simulink model "Modular_Model_New_Board"  (R2018a)
settings: Solver=FixedStepAuto  StartTime=0.0  StopTime=Tfinal  FixedStep=SampleTime*1e-2  MinStep=SampleTime*1e-2  RelTol=1e-3
values from neighbouring files (symbols this model uses):
  ESRA = 21.1e-3    (= 0.0211)    [sim_param_new_board.m]
  ESRB = 21.1e-3    (= 0.0211)    [sim_param_new_board.m]
  ESRC = 21.1e-3    (= 0.0211)    [sim_param_new_board.m]
  ffund = 50    [sim_param_new_board.m]
  LAMid = 01.30e-9    (= 1.3e-09)    [sim_param_new_board.m]
  LBMid = 01.30e-9    (= 1.3e-09)    [sim_param_new_board.m]
  LCMid = 01.30e-9    (= 1.3e-09)    [sim_param_new_board.m]
  ModulationIndex1 = 0.9    [sim_param_new_board.m]
  Module1Phase = 0    [sim_param_new_board.m]
  RABBot = 10.20e-9    (= 1.02e-08)    [sim_param_new_board.m]
  RABot = 20.25e-9    (= 2.025e-08)    [sim_param_new_board.m]
  RABTop = 18.30e-9    (= 1.83e-08)    [sim_param_new_board.m]
  RAMid = 01.30e-9    (= 1.3e-09)    [sim_param_new_board.m]
  RATop = 03.40e-9    (= 3.4e-09)    [sim_param_new_board.m]
  RBBot = 20.38e-9    (= 2.038e-08)    [sim_param_new_board.m]
  RBCBot = 11.14e-9    (= 1.114e-08)    [sim_param_new_board.m]
  RBCTop = 21.84e-9    (= 2.184e-08)    [sim_param_new_board.m]
  RBMid = 01.30e-9    (= 1.3e-09)    [sim_param_new_board.m]
  RBTop = 03.38e-9    (= 3.38e-09)    [sim_param_new_board.m]
  RCBot = 20.94e-9    (= 2.094e-08)    [sim_param_new_board.m]
  RCMid = 01.30e-9    (= 1.3e-09)    [sim_param_new_board.m]
  RCTop = 03.41e-9    (= 3.41e-09)    [sim_param_new_board.m]
  Rin = 0.1    [sim_param_new_board.m]
  Rload1 = Z1*PF    [sim_param_new_board.m]
  Vmodule = 270    [sim_param_new_board.m]
  VpulseMax = 6    [sim_param_new_board.m]
  VpulseMin = -3    [sim_param_new_board.m]
libraries: elec_lib x81, fl_lib x38, nesl_utility x38, simulink x12, powerlib_meascontrol x4
(part 3 of 3)

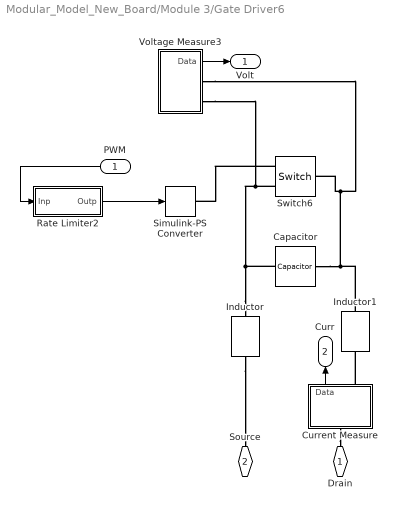
== system Modular_Model_New_Board/Module 3/Gate Driver6 ==
  PWM : Inport
  Capacitor : elec_lib/Passive Devices/Capacitor  enable_table=0  c=142e-12 F  Cvec=[1e-05, 1e-06] F  Vvec=[0, 10] V  CV_table_symmetry=1  C_tol=5  enable_C_tol=0  tol_distribution=1  nSigma=4  r=1e-6 Ohm  g=0 1/Ohm  enable_operating_limits=0  operating_limit_action=2  max_working_voltage_range=[-25, 25] V  power_rating=1 W  enable_faults=0  fault_action=1  Cscale_faulted=100  R_faulted=1e-3 Ohm  G_faulted=0 1/Ohm  tau_fault=1e-3 s  enable_temporal_fault=0  t_fault=1 s  enable_behavioral_fault=0  max_permissible_voltage_range=[-100, 100] V  t_fail_on_voltage=1 s  i_specify=off  i_priority=None  i=0 A  i_nominal_specify=off  i_nominal_unit=A  i_nominal_value=1  v_specify=off  v_priority=None  v=0 V  v_nominal_specify=off  v_nominal_unit=V  v_nominal_value=1  vc_specify=on  vc_priority=High  vc=0 V  vc_nominal_specify=off  vc_nominal_unit=V  vc_nominal_value=1
  Current Measure : Subsystem
  Inductor : elec_lib/Passive Devices/Inductor  l=Ls H  L_tol=20  enable_L_tol=0  tol_distribution=1  nSigma=4  r=0 Ohm  g=1e-9 1/Ohm  enable_operating_limits=0  operating_limit_action=2  max_working_current=1 A  power_rating=1 W  enable_faults=0  fault_action=1  lambdaPercent=50  k_faulted=0.9999  turnsShort=0  openCct=0  groundShort=0  groundShortG=0 1/Ohm  tau_fault=1e-3 s  enable_temporal_fault=0  t_fault=1 s  enable_behavioral_fault=0  max_permissible_voltage=100 V  n_fail_on_voltage=1  max_permissible_current=1 A  t_fail_on_current=1 s  i_L_specify=on  i_L_priority=High  i_L=0 A  i_L_nominal_specify=off  i_L_nominal_unit=A  i_L_nominal_value=1
      settings: SourceProductName=Simscape Electronics  SourceProductBaseCode=SN
  Inductor1 : elec_lib/Passive Devices/Inductor  l=Ld H  L_tol=20  enable_L_tol=0  tol_distribution=1  nSigma=4  r=0 Ohm  g=1e-9 1/Ohm  enable_operating_limits=0  operating_limit_action=2  max_working_current=1 A  power_rating=1 W  enable_faults=0  fault_action=1  lambdaPercent=50  k_faulted=0.9999  turnsShort=0  openCct=0  groundShort=0  groundShortG=0 1/Ohm  tau_fault=1e-3 s  enable_temporal_fault=0  t_fault=1 s  enable_behavioral_fault=0  max_permissible_voltage=100 V  n_fail_on_voltage=1  max_permissible_current=1 A  t_fail_on_current=1 s  i_L_specify=on  i_L_priority=High  i_L=0 A  i_L_nominal_specify=off  i_L_nominal_unit=A  i_L_nominal_value=1
      settings: SourceProductName=Simscape Electronics  SourceProductBaseCode=SN
  Rate Limiter2 : Subsystem
  Simulink-PS Converter : nesl_utility/Simulink-PS Converter  PhysicalDomain=network_engine_domain  SubClassName=ps_input  LeftPortType=input  RightPortType=output  PseudoPeriodic=off  Frequencies=[]  NoiseDistribution=none  NoiseParameters=[]  Unit=1  AffineConversion=off  FilteringAndDerivatives=zero  SimscapeFilterOrder=1  InputFilterTimeConstant=0.001  UdotUserProvided=1
  Switch6 : fl_lib/Electrical/Electrical Elements/Switch  R_closed=0.05 Ohm  G_open=1e-8 1/Ohm  Threshold=1.7  i_specify=off  i_priority=None  i=0 A  i_nominal_specify=off  i_nominal_unit=A  i_nominal_value=1  v_specify=off  v_priority=None  v=0 V  v_nominal_specify=off  v_nominal_unit=V  v_nominal_value=1
      settings: SourceProductName=Simscape
  Voltage Measure3 : Subsystem
  Drain : PMIOPort  Side=Left
  Source : PMIOPort  Port=2  Side=Left
  Volt : Outport
  Curr : Outport  Port=2
  wires:
  PWM/1 -> Rate Limiter2/1(Inp)
  Rate Limiter2/1(Outp) -> Simulink-PS Converter/1
  Voltage Measure3/1(Data) -> Volt/1
  Current Measure/1(Data) -> Curr/1
  connections:
  Switch6/RConn1 -- Simulink-PS Converter/RConn1
  Inductor/LConn1 -- Voltage Measure3/RConn2 -- Switch6/RConn2 -- Capacitor/RConn1
  Voltage Measure3/RConn1 -- Switch6/LConn1 -- Capacitor/LConn1 -- Inductor1/LConn1
  Current Measure/LConn1 -- Drain/RConn1
  Inductor/RConn1 -- Source/RConn1
  Current Measure/RConn1 -- Inductor1/RConn1

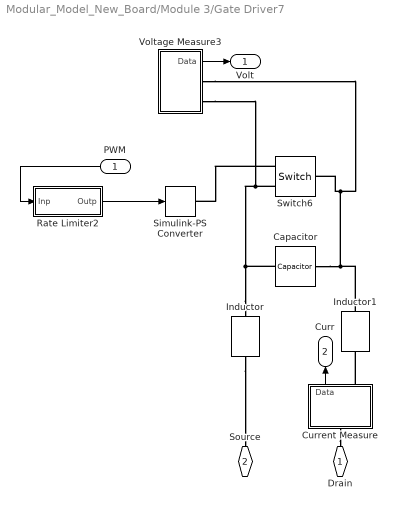
== system Modular_Model_New_Board/Module 3/Gate Driver7 ==
  PWM : Inport
  Capacitor : elec_lib/Passive Devices/Capacitor  enable_table=0  c=142e-12 F  Cvec=[1e-05, 1e-06] F  Vvec=[0, 10] V  CV_table_symmetry=1  C_tol=5  enable_C_tol=0  tol_distribution=1  nSigma=4  r=1e-6 Ohm  g=0 1/Ohm  enable_operating_limits=0  operating_limit_action=2  max_working_voltage_range=[-25, 25] V  power_rating=1 W  enable_faults=0  fault_action=1  Cscale_faulted=100  R_faulted=1e-3 Ohm  G_faulted=0 1/Ohm  tau_fault=1e-3 s  enable_temporal_fault=0  t_fault=1 s  enable_behavioral_fault=0  max_permissible_voltage_range=[-100, 100] V  t_fail_on_voltage=1 s  i_specify=off  i_priority=None  i=0 A  i_nominal_specify=off  i_nominal_unit=A  i_nominal_value=1  v_specify=off  v_priority=None  v=0 V  v_nominal_specify=off  v_nominal_unit=V  v_nominal_value=1  vc_specify=on  vc_priority=High  vc=0 V  vc_nominal_specify=off  vc_nominal_unit=V  vc_nominal_value=1
  Current Measure : Subsystem
  Inductor : elec_lib/Passive Devices/Inductor  l=Ls H  L_tol=20  enable_L_tol=0  tol_distribution=1  nSigma=4  r=0 Ohm  g=1e-9 1/Ohm  enable_operating_limits=0  operating_limit_action=2  max_working_current=1 A  power_rating=1 W  enable_faults=0  fault_action=1  lambdaPercent=50  k_faulted=0.9999  turnsShort=0  openCct=0  groundShort=0  groundShortG=0 1/Ohm  tau_fault=1e-3 s  enable_temporal_fault=0  t_fault=1 s  enable_behavioral_fault=0  max_permissible_voltage=100 V  n_fail_on_voltage=1  max_permissible_current=1 A  t_fail_on_current=1 s  i_L_specify=on  i_L_priority=High  i_L=0 A  i_L_nominal_specify=off  i_L_nominal_unit=A  i_L_nominal_value=1
      settings: SourceProductName=Simscape Electronics  SourceProductBaseCode=SN
  Inductor1 : elec_lib/Passive Devices/Inductor  l=Ld H  L_tol=20  enable_L_tol=0  tol_distribution=1  nSigma=4  r=0 Ohm  g=1e-9 1/Ohm  enable_operating_limits=0  operating_limit_action=2  max_working_current=1 A  power_rating=1 W  enable_faults=0  fault_action=1  lambdaPercent=50  k_faulted=0.9999  turnsShort=0  openCct=0  groundShort=0  groundShortG=0 1/Ohm  tau_fault=1e-3 s  enable_temporal_fault=0  t_fault=1 s  enable_behavioral_fault=0  max_permissible_voltage=100 V  n_fail_on_voltage=1  max_permissible_current=1 A  t_fail_on_current=1 s  i_L_specify=on  i_L_priority=High  i_L=0 A  i_L_nominal_specify=off  i_L_nominal_unit=A  i_L_nominal_value=1
      settings: SourceProductName=Simscape Electronics  SourceProductBaseCode=SN
  Rate Limiter2 : Subsystem
  Simulink-PS Converter : nesl_utility/Simulink-PS Converter  PhysicalDomain=network_engine_domain  SubClassName=ps_input  LeftPortType=input  RightPortType=output  PseudoPeriodic=off  Frequencies=[]  NoiseDistribution=none  NoiseParameters=[]  Unit=1  AffineConversion=off  FilteringAndDerivatives=zero  SimscapeFilterOrder=1  InputFilterTimeConstant=0.001  UdotUserProvided=1
  Switch6 : fl_lib/Electrical/Electrical Elements/Switch  R_closed=0.05 Ohm  G_open=1e-8 1/Ohm  Threshold=1.7  i_specify=off  i_priority=None  i=0 A  i_nominal_specify=off  i_nominal_unit=A  i_nominal_value=1  v_specify=off  v_priority=None  v=0 V  v_nominal_specify=off  v_nominal_unit=V  v_nominal_value=1
      settings: SourceProductName=Simscape
  Voltage Measure3 : Subsystem
  Drain : PMIOPort  Side=Left
  Source : PMIOPort  Port=2  Side=Left
  Volt : Outport
  Curr : Outport  Port=2
  wires:
  PWM/1 -> Rate Limiter2/1(Inp)
  Rate Limiter2/1(Outp) -> Simulink-PS Converter/1
  Voltage Measure3/1(Data) -> Volt/1
  Current Measure/1(Data) -> Curr/1
  connections:
  Switch6/RConn1 -- Simulink-PS Converter/RConn1
  Inductor/LConn1 -- Voltage Measure3/RConn2 -- Switch6/RConn2 -- Capacitor/RConn1
  Voltage Measure3/RConn1 -- Switch6/LConn1 -- Capacitor/LConn1 -- Inductor1/LConn1
  Current Measure/LConn1 -- Drain/RConn1
  Inductor/RConn1 -- Source/RConn1
  Current Measure/RConn1 -- Inductor1/RConn1

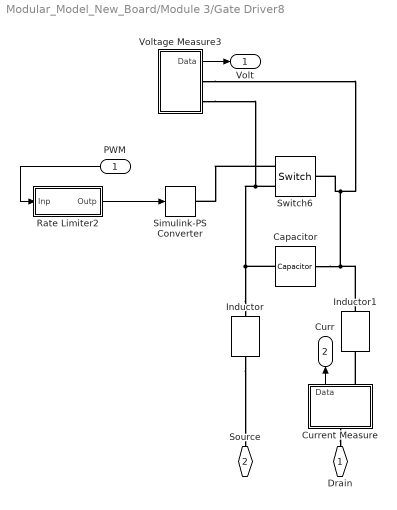
== system Modular_Model_New_Board/Module 3/Gate Driver8 ==
  PWM : Inport
  Capacitor : elec_lib/Passive Devices/Capacitor  enable_table=0  c=142e-12 F  Cvec=[1e-05, 1e-06] F  Vvec=[0, 10] V  CV_table_symmetry=1  C_tol=5  enable_C_tol=0  tol_distribution=1  nSigma=4  r=1e-6 Ohm  g=0 1/Ohm  enable_operating_limits=0  operating_limit_action=2  max_working_voltage_range=[-25, 25] V  power_rating=1 W  enable_faults=0  fault_action=1  Cscale_faulted=100  R_faulted=1e-3 Ohm  G_faulted=0 1/Ohm  tau_fault=1e-3 s  enable_temporal_fault=0  t_fault=1 s  enable_behavioral_fault=0  max_permissible_voltage_range=[-100, 100] V  t_fail_on_voltage=1 s  i_specify=off  i_priority=None  i=0 A  i_nominal_specify=off  i_nominal_unit=A  i_nominal_value=1  v_specify=off  v_priority=None  v=0 V  v_nominal_specify=off  v_nominal_unit=V  v_nominal_value=1  vc_specify=on  vc_priority=High  vc=0 V  vc_nominal_specify=off  vc_nominal_unit=V  vc_nominal_value=1
  Current Measure : Subsystem
  Inductor : elec_lib/Passive Devices/Inductor  l=Ls H  L_tol=20  enable_L_tol=0  tol_distribution=1  nSigma=4  r=0 Ohm  g=1e-9 1/Ohm  enable_operating_limits=0  operating_limit_action=2  max_working_current=1 A  power_rating=1 W  enable_faults=0  fault_action=1  lambdaPercent=50  k_faulted=0.9999  turnsShort=0  openCct=0  groundShort=0  groundShortG=0 1/Ohm  tau_fault=1e-3 s  enable_temporal_fault=0  t_fault=1 s  enable_behavioral_fault=0  max_permissible_voltage=100 V  n_fail_on_voltage=1  max_permissible_current=1 A  t_fail_on_current=1 s  i_L_specify=on  i_L_priority=High  i_L=0 A  i_L_nominal_specify=off  i_L_nominal_unit=A  i_L_nominal_value=1
      settings: SourceProductName=Simscape Electronics  SourceProductBaseCode=SN
  Inductor1 : elec_lib/Passive Devices/Inductor  l=Ld H  L_tol=20  enable_L_tol=0  tol_distribution=1  nSigma=4  r=0 Ohm  g=1e-9 1/Ohm  enable_operating_limits=0  operating_limit_action=2  max_working_current=1 A  power_rating=1 W  enable_faults=0  fault_action=1  lambdaPercent=50  k_faulted=0.9999  turnsShort=0  openCct=0  groundShort=0  groundShortG=0 1/Ohm  tau_fault=1e-3 s  enable_temporal_fault=0  t_fault=1 s  enable_behavioral_fault=0  max_permissible_voltage=100 V  n_fail_on_voltage=1  max_permissible_current=1 A  t_fail_on_current=1 s  i_L_specify=on  i_L_priority=High  i_L=0 A  i_L_nominal_specify=off  i_L_nominal_unit=A  i_L_nominal_value=1
      settings: SourceProductName=Simscape Electronics  SourceProductBaseCode=SN
  Rate Limiter2 : Subsystem
  Simulink-PS Converter : nesl_utility/Simulink-PS Converter  PhysicalDomain=network_engine_domain  SubClassName=ps_input  LeftPortType=input  RightPortType=output  PseudoPeriodic=off  Frequencies=[]  NoiseDistribution=none  NoiseParameters=[]  Unit=1  AffineConversion=off  FilteringAndDerivatives=zero  SimscapeFilterOrder=1  InputFilterTimeConstant=0.001  UdotUserProvided=1
  Switch6 : fl_lib/Electrical/Electrical Elements/Switch  R_closed=0.05 Ohm  G_open=1e-8 1/Ohm  Threshold=1.7  i_specify=off  i_priority=None  i=0 A  i_nominal_specify=off  i_nominal_unit=A  i_nominal_value=1  v_specify=off  v_priority=None  v=0 V  v_nominal_specify=off  v_nominal_unit=V  v_nominal_value=1
      settings: SourceProductName=Simscape
  Voltage Measure3 : Subsystem
  Drain : PMIOPort  Side=Left
  Source : PMIOPort  Port=2  Side=Left
  Volt : Outport
  Curr : Outport  Port=2
  wires:
  PWM/1 -> Rate Limiter2/1(Inp)
  Rate Limiter2/1(Outp) -> Simulink-PS Converter/1
  Voltage Measure3/1(Data) -> Volt/1
  Current Measure/1(Data) -> Curr/1
  connections:
  Switch6/RConn1 -- Simulink-PS Converter/RConn1
  Inductor/LConn1 -- Voltage Measure3/RConn2 -- Switch6/RConn2 -- Capacitor/RConn1
  Voltage Measure3/RConn1 -- Switch6/LConn1 -- Capacitor/LConn1 -- Inductor1/LConn1
  Current Measure/LConn1 -- Drain/RConn1
  Inductor/RConn1 -- Source/RConn1
  Current Measure/RConn1 -- Inductor1/RConn1

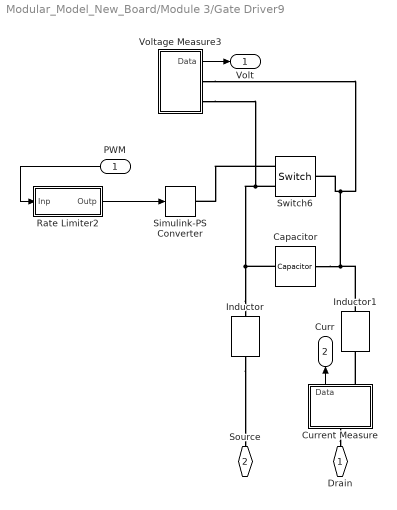
== system Modular_Model_New_Board/Module 3/Gate Driver9 ==
  PWM : Inport
  Capacitor : elec_lib/Passive Devices/Capacitor  enable_table=0  c=142e-12 F  Cvec=[1e-05, 1e-06] F  Vvec=[0, 10] V  CV_table_symmetry=1  C_tol=5  enable_C_tol=0  tol_distribution=1  nSigma=4  r=1e-6 Ohm  g=0 1/Ohm  enable_operating_limits=0  operating_limit_action=2  max_working_voltage_range=[-25, 25] V  power_rating=1 W  enable_faults=0  fault_action=1  Cscale_faulted=100  R_faulted=1e-3 Ohm  G_faulted=0 1/Ohm  tau_fault=1e-3 s  enable_temporal_fault=0  t_fault=1 s  enable_behavioral_fault=0  max_permissible_voltage_range=[-100, 100] V  t_fail_on_voltage=1 s  i_specify=off  i_priority=None  i=0 A  i_nominal_specify=off  i_nominal_unit=A  i_nominal_value=1  v_specify=off  v_priority=None  v=0 V  v_nominal_specify=off  v_nominal_unit=V  v_nominal_value=1  vc_specify=on  vc_priority=High  vc=0 V  vc_nominal_specify=off  vc_nominal_unit=V  vc_nominal_value=1
  Current Measure : Subsystem
  Inductor : elec_lib/Passive Devices/Inductor  l=Ls H  L_tol=20  enable_L_tol=0  tol_distribution=1  nSigma=4  r=0 Ohm  g=1e-9 1/Ohm  enable_operating_limits=0  operating_limit_action=2  max_working_current=1 A  power_rating=1 W  enable_faults=0  fault_action=1  lambdaPercent=50  k_faulted=0.9999  turnsShort=0  openCct=0  groundShort=0  groundShortG=0 1/Ohm  tau_fault=1e-3 s  enable_temporal_fault=0  t_fault=1 s  enable_behavioral_fault=0  max_permissible_voltage=100 V  n_fail_on_voltage=1  max_permissible_current=1 A  t_fail_on_current=1 s  i_L_specify=on  i_L_priority=High  i_L=0 A  i_L_nominal_specify=off  i_L_nominal_unit=A  i_L_nominal_value=1
      settings: SourceProductName=Simscape Electronics  SourceProductBaseCode=SN
  Inductor1 : elec_lib/Passive Devices/Inductor  l=Ld H  L_tol=20  enable_L_tol=0  tol_distribution=1  nSigma=4  r=0 Ohm  g=1e-9 1/Ohm  enable_operating_limits=0  operating_limit_action=2  max_working_current=1 A  power_rating=1 W  enable_faults=0  fault_action=1  lambdaPercent=50  k_faulted=0.9999  turnsShort=0  openCct=0  groundShort=0  groundShortG=0 1/Ohm  tau_fault=1e-3 s  enable_temporal_fault=0  t_fault=1 s  enable_behavioral_fault=0  max_permissible_voltage=100 V  n_fail_on_voltage=1  max_permissible_current=1 A  t_fail_on_current=1 s  i_L_specify=on  i_L_priority=High  i_L=0 A  i_L_nominal_specify=off  i_L_nominal_unit=A  i_L_nominal_value=1
      settings: SourceProductName=Simscape Electronics  SourceProductBaseCode=SN
  Rate Limiter2 : Subsystem
  Simulink-PS Converter : nesl_utility/Simulink-PS Converter  PhysicalDomain=network_engine_domain  SubClassName=ps_input  LeftPortType=input  RightPortType=output  PseudoPeriodic=off  Frequencies=[]  NoiseDistribution=none  NoiseParameters=[]  Unit=1  AffineConversion=off  FilteringAndDerivatives=zero  SimscapeFilterOrder=1  InputFilterTimeConstant=0.001  UdotUserProvided=1
  Switch6 : fl_lib/Electrical/Electrical Elements/Switch  R_closed=0.05 Ohm  G_open=1e-8 1/Ohm  Threshold=1.7  i_specify=off  i_priority=None  i=0 A  i_nominal_specify=off  i_nominal_unit=A  i_nominal_value=1  v_specify=off  v_priority=None  v=0 V  v_nominal_specify=off  v_nominal_unit=V  v_nominal_value=1
      settings: SourceProductName=Simscape
  Voltage Measure3 : Subsystem
  Drain : PMIOPort  Side=Left
  Source : PMIOPort  Port=2  Side=Left
  Volt : Outport
  Curr : Outport  Port=2
  wires:
  PWM/1 -> Rate Limiter2/1(Inp)
  Rate Limiter2/1(Outp) -> Simulink-PS Converter/1
  Voltage Measure3/1(Data) -> Volt/1
  Current Measure/1(Data) -> Curr/1
  connections:
  Switch6/RConn1 -- Simulink-PS Converter/RConn1
  Inductor/LConn1 -- Voltage Measure3/RConn2 -- Switch6/RConn2 -- Capacitor/RConn1
  Voltage Measure3/RConn1 -- Switch6/LConn1 -- Capacitor/LConn1 -- Inductor1/LConn1
  Current Measure/LConn1 -- Drain/RConn1
  Inductor/RConn1 -- Source/RConn1
  Current Measure/RConn1 -- Inductor1/RConn1

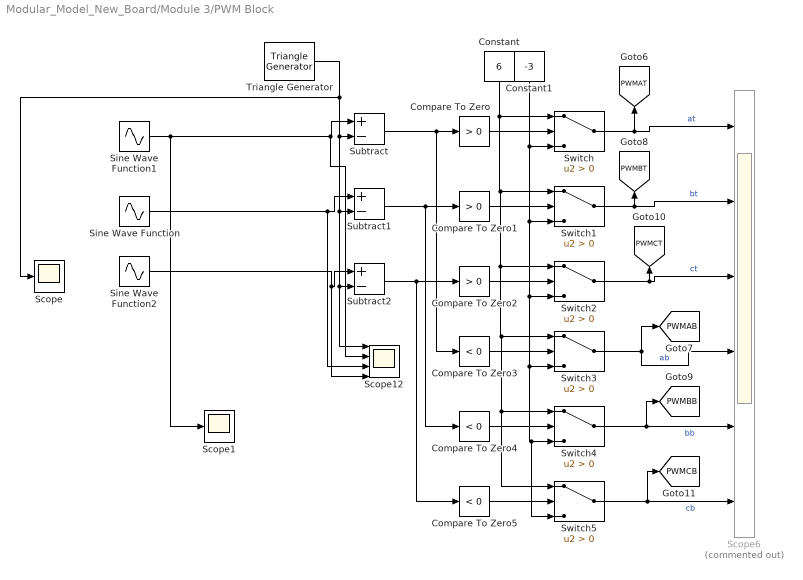
== system Modular_Model_New_Board/Module 3/PWM Block ==
  Compare To Zero : simulink/Logic and Bit Operations/Compare To Zero  relop=>  OutDataTypeStr=boolean
  Compare To Zero1 : simulink/Logic and Bit Operations/Compare To Zero  relop=>  OutDataTypeStr=boolean
  Compare To Zero2 : simulink/Logic and Bit Operations/Compare To Zero  relop=>  OutDataTypeStr=boolean
  Compare To Zero3 : simulink/Logic and Bit Operations/Compare To Zero  relop=<  OutDataTypeStr=boolean
  Compare To Zero4 : simulink/Logic and Bit Operations/Compare To Zero  relop=<  OutDataTypeStr=boolean
  Compare To Zero5 : simulink/Logic and Bit Operations/Compare To Zero  relop=<  OutDataTypeStr=boolean
  Constant : Constant  Value=6
  Constant1 : Constant  Value=-3
  Scope : Scope
  Scope1 : Scope
  Scope12 : Scope  NumInputPorts=4
  Scope6 : Scope  Commented=on  NumInputPorts=6
  Sine Wave Function : Sin  Amplitude=ModulationIndex1  Frequency=ffund*2*pi  Phase=-2*pi/3  SampleTime=0
  Sine Wave Function1 : Sin  Amplitude=ModulationIndex1  Frequency=ffund*2*pi  SampleTime=0
  Sine Wave Function2 : Sin  Amplitude=ModulationIndex1  Frequency=ffund*2*pi  Phase=2*pi/3  SampleTime=0
  Subtract : Sum  Inputs=+-
  Subtract1 : Sum  Inputs=+-
  Subtract2 : Sum  Inputs=+-
  Switch{,1..5} (6 alike) : Switch  Criteria=u2 > Threshold
  Triangle Generator : powerlib_meascontrol/Pulse & Signal Generators/Triangle Generator  Freq=fsw  Phase=Module1Phase  Ts=0
  tag scope: PWMAB=global, PWMAT=global, PWMBB=global, PWMBT=global, PWMCB=global, PWMCT=global
  wires:
  Switch2/1 -> [PWMCT], Scope6/3  "ct"
  Constant/1 -> Switch5/1, Switch4/1, Switch3/1, Switch2/1, Switch1/1, Switch/1
  Sine Wave Function/1 -> Subtract1/1, Scope12/3
  Subtract2/1 -> Compare To Zero5/1, Compare To Zero2/1
  Compare To Zero/1 -> Switch/2
  Sine Wave Function1/1 -> Scope1/1, Scope12/2, Subtract/1
  Compare To Zero1/1 -> Switch1/2
  Constant1/1 -> Switch/3, Switch1/3, Switch5/3, Switch4/3, Switch3/3, Switch2/3
  Subtract1/1 -> Compare To Zero4/1, Compare To Zero1/1
  Triangle Generator/1 -> Scope/1, Scope12/1, Subtract2/2, Subtract1/2, Subtract/2
  Switch/1 -> [PWMAT], Scope6/1  "at"
  Subtract/1 -> Compare To Zero3/1, Compare To Zero/1
  Switch1/1 -> [PWMBT], Scope6/2  "bt"
  Switch5/1 -> [PWMCB], Scope6/6  "cb"
  Compare To Zero5/1 -> Switch5/2
  Compare To Zero4/1 -> Switch4/2
  Compare To Zero3/1 -> Switch3/2
  Switch4/1 -> [PWMBB], Scope6/5  "bb"
  Sine Wave Function2/1 -> Scope12/4, Subtract2/1
  Compare To Zero2/1 -> Switch2/2
  Switch3/1 -> [PWMAB], Scope6/4  "ab"

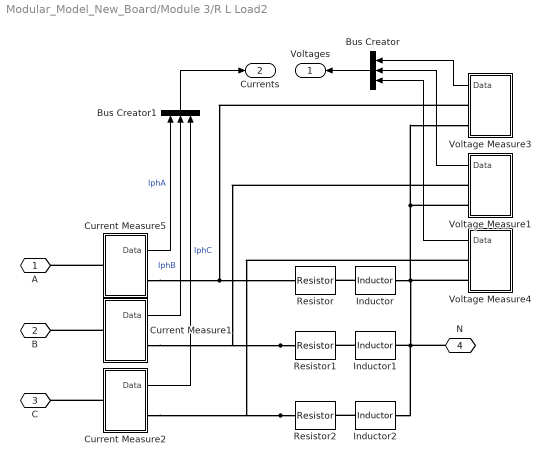
== system Modular_Model_New_Board/Module 3/R L Load2 ==
  Bus Creator : BusCreator  Inputs=3
  Bus Creator1 : BusCreator  Inputs=3
  Current Measure1 : Subsystem
  Current Measure2 : Subsystem
  Current Measure5 : Subsystem
  Inductor : elec_lib/Passive Devices/Inductor  l=Lload1 H  L_tol=20  enable_L_tol=0  tol_distribution=1  nSigma=4  r=0 Ohm  g=1e-9 1/Ohm  enable_operating_limits=0  operating_limit_action=2  max_working_current=1 A  power_rating=1 W  enable_faults=0  fault_action=1  lambdaPercent=50  k_faulted=0.9999  turnsShort=0  openCct=0  groundShort=0  groundShortG=0 1/Ohm  tau_fault=0.001 s  enable_temporal_fault=0  t_fault=1 s  enable_behavioral_fault=0  max_permissible_voltage=100 V  n_fail_on_voltage=1  max_permissible_current=1 A  t_fail_on_current=1 s  i_L_specify=on  i_L_priority=High  i_L=0 A  i_L_nominal_specify=off  i_L_nominal_unit=A  i_L_nominal_value=1
      settings: SourceProductName=Simscape Electronics  SourceProductBaseCode=SN
  Inductor1 : elec_lib/Passive Devices/Inductor  l=Lload1 H  L_tol=20  enable_L_tol=0  tol_distribution=1  nSigma=4  r=0 Ohm  g=1e-9 1/Ohm  enable_operating_limits=0  operating_limit_action=2  max_working_current=1 A  power_rating=1 W  enable_faults=0  fault_action=1  lambdaPercent=50  k_faulted=0.9999  turnsShort=0  openCct=0  groundShort=0  groundShortG=0 1/Ohm  tau_fault=0.001 s  enable_temporal_fault=0  t_fault=1 s  enable_behavioral_fault=0  max_permissible_voltage=100 V  n_fail_on_voltage=1  max_permissible_current=1 A  t_fail_on_current=1 s  i_L_specify=on  i_L_priority=High  i_L=0 A  i_L_nominal_specify=off  i_L_nominal_unit=A  i_L_nominal_value=1
      settings: SourceProductName=Simscape Electronics  SourceProductBaseCode=SN
  Inductor2 : elec_lib/Passive Devices/Inductor  l=Lload1 H  L_tol=20  enable_L_tol=0  tol_distribution=1  nSigma=4  r=0 Ohm  g=1e-9 1/Ohm  enable_operating_limits=0  operating_limit_action=2  max_working_current=1 A  power_rating=1 W  enable_faults=0  fault_action=1  lambdaPercent=50  k_faulted=0.9999  turnsShort=0  openCct=0  groundShort=0  groundShortG=0 1/Ohm  tau_fault=0.001 s  enable_temporal_fault=0  t_fault=1 s  enable_behavioral_fault=0  max_permissible_voltage=100 V  n_fail_on_voltage=1  max_permissible_current=1 A  t_fail_on_current=1 s  i_L_specify=on  i_L_priority=High  i_L=0 A  i_L_nominal_specify=off  i_L_nominal_unit=A  i_L_nominal_value=1
      settings: SourceProductName=Simscape Electronics  SourceProductBaseCode=SN
  Resistor : elec_lib/Passive Devices/Resistor  R=Rload1 Ohm  R_tol=5  enable_R_tol=0  tol_distribution=1  nSigma=4  enable_operating_limits=0  operating_limit_action=2  max_working_voltage=100 V  power_rating=1 W  enable_faults=0  fault_action=1  R_faulted=Inf Ohm  enable_temporal_fault=0  t_fault=1 s  enable_behavioral_fault=0  max_permissible_current=1 A  t_fail_on_current=1 s  noise_mode=0  sample_time=0.001 s  repeatability=1  auto_seed=1554434926  user_seed=0  Tdevice=25 degC  alpha=3.93e-3 1/K  Tmeas=25 degC  thermal_mass=100 J/K  power_derating_T1=70 degC  power_derating_T2=155 degC  operating_temperature_range_vec=[-50, 150] degC  temperature_specify=off  temperature_priority=High  temperature=298.15 K  temperature_nominal_specify=off  temperature_nominal_unit=K  temperature_nominal_value=1
  Resistor1 : elec_lib/Passive Devices/Resistor  R=Rload1 Ohm  R_tol=5  enable_R_tol=0  tol_distribution=1  nSigma=4  enable_operating_limits=0  operating_limit_action=2  max_working_voltage=100 V  power_rating=1 W  enable_faults=0  fault_action=1  R_faulted=Inf Ohm  enable_temporal_fault=0  t_fault=1 s  enable_behavioral_fault=0  max_permissible_current=1 A  t_fail_on_current=1 s  noise_mode=0  sample_time=0.001 s  repeatability=1  auto_seed=3113098355  user_seed=0  Tdevice=25 degC  alpha=3.93e-3 1/K  Tmeas=25 degC  thermal_mass=100 J/K  power_derating_T1=70 degC  power_derating_T2=155 degC  operating_temperature_range_vec=[-50, 150] degC  temperature_specify=off  temperature_priority=High  temperature=298.15 K  temperature_nominal_specify=off  temperature_nominal_unit=K  temperature_nominal_value=1
  Resistor2 : elec_lib/Passive Devices/Resistor  R=Rload1 Ohm  R_tol=5  enable_R_tol=0  tol_distribution=1  nSigma=4  enable_operating_limits=0  operating_limit_action=2  max_working_voltage=100 V  power_rating=1 W  enable_faults=0  fault_action=1  R_faulted=Inf Ohm  enable_temporal_fault=0  t_fault=1 s  enable_behavioral_fault=0  max_permissible_current=1 A  t_fail_on_current=1 s  noise_mode=0  sample_time=0.001 s  repeatability=1  auto_seed=3686420587  user_seed=0  Tdevice=25 degC  alpha=3.93e-3 1/K  Tmeas=25 degC  thermal_mass=100 J/K  power_derating_T1=70 degC  power_derating_T2=155 degC  operating_temperature_range_vec=[-50, 150] degC  temperature_specify=off  temperature_priority=High  temperature=298.15 K  temperature_nominal_specify=off  temperature_nominal_unit=K  temperature_nominal_value=1
  Voltage Measure1 : Subsystem
  Voltage Measure3 : Subsystem
  Voltage Measure4 : Subsystem
  A : PMIOPort  Side=Left
  B : PMIOPort  Port=2  Side=Left
  C : PMIOPort  Port=3  Side=Left
  N : PMIOPort  Port=4  Side=Right
  Voltages : Outport
  Currents : Outport  Port=2
  wires:
  Current Measure5/1(Data) -> Bus Creator1/1  "IphA"
  Current Measure1/1(Data) -> Bus Creator1/2  "IphB"
  Current Measure2/1(Data) -> Bus Creator1/3  "IphC"
  Bus Creator/1 -> Voltages/1
  Bus Creator1/1 -> Currents/1
  Voltage Measure3/1(Data) -> Bus Creator/1
  Voltage Measure1/1(Data) -> Bus Creator/2
  Voltage Measure4/1(Data) -> Bus Creator/3
  connections:
  Inductor/LConn1 -- Resistor/RConn1
  Voltage Measure4/RConn2 -- Inductor/RConn1 -- Voltage Measure1/RConn2 -- Voltage Measure3/RConn2 -- Inductor2/RConn1 -- Inductor1/RConn1 -- N/RConn1
  Inductor2/LConn1 -- Resistor2/RConn1
  Inductor1/LConn1 -- Resistor1/RConn1
  Resistor1/LConn1 -- Current Measure1/RConn1 -- Voltage Measure1/RConn1
  Voltage Measure3/RConn1 -- Current Measure5/RConn1 -- Resistor/LConn1
  Current Measure5/LConn1 -- A/RConn1
  Current Measure1/LConn1 -- B/RConn1
  Current Measure2/LConn1 -- C/RConn1
  Resistor2/LConn1 -- Current Measure2/RConn1 -- Voltage Measure4/RConn1

== system Modular_Model_New_Board/Module 3/Subsystem ==
  Current Sensor2 : fl_lib/Electrical/Electrical Sensors/Current Sensor
  PS-Simulink Converter3 : nesl_utility/PS-Simulink Converter  PhysicalDomain=network_engine_domain  SubClassName=ps_output  LeftPortType=input  RightPortType=output  PseudoPeriodic=off  Frequencies=[]  Unit=1  AffineConversion=off
  + : PMIOPort  Side=Left
  - : PMIOPort  Port=2  Side=Right
  tag scope: ACapCurr=global
  wires:
  PS-Simulink Converter3/1 -> [ACapCurr]
  connections:
  Current Sensor2/RConn2 -- -/RConn1
  PS-Simulink Converter3/LConn1 -- Current Sensor2/RConn1
  Current Sensor2/LConn1 -- +/RConn1

== system Modular_Model_New_Board/Module 3/Subsystem1 ==
  PS-Simulink Converter1 : nesl_utility/PS-Simulink Converter  PhysicalDomain=network_engine_domain  SubClassName=ps_output  LeftPortType=input  RightPortType=output  PseudoPeriodic=off  Frequencies=[]  Unit=1  AffineConversion=off
  Voltage Sensor1 : fl_lib/Electrical/Electrical Sensors/Voltage Sensor
  + : PMIOPort  Side=Left
  - : PMIOPort  Port=2  Side=Right
  tag scope: ACap=global
  wires:
  PS-Simulink Converter1/1 -> [ACap]
  connections:
  PS-Simulink Converter1/LConn1 -- Voltage Sensor1/RConn1
  Voltage Sensor1/RConn2 -- -/RConn1
  Voltage Sensor1/LConn1 -- +/RConn1

== system Modular_Model_New_Board/Module 3/Subsystem2 ==
  Current Sensor3 : fl_lib/Electrical/Electrical Sensors/Current Sensor
  PS-Simulink Converter5 : nesl_utility/PS-Simulink Converter  PhysicalDomain=network_engine_domain  SubClassName=ps_output  LeftPortType=input  RightPortType=output  PseudoPeriodic=off  Frequencies=[]  Unit=1  AffineConversion=off
  + : PMIOPort  Side=Left
  - : PMIOPort  Port=2  Side=Right
  tag scope: BCapCurr=global
  wires:
  PS-Simulink Converter5/1 -> [BCapCurr]
  connections:
  PS-Simulink Converter5/LConn1 -- Current Sensor3/RConn1
  Current Sensor3/RConn2 -- -/RConn1
  Current Sensor3/LConn1 -- +/RConn1

== system Modular_Model_New_Board/Module 3/Subsystem3 ==
  PS-Simulink Converter7 : nesl_utility/PS-Simulink Converter  PhysicalDomain=network_engine_domain  SubClassName=ps_output  LeftPortType=input  RightPortType=output  PseudoPeriodic=off  Frequencies=[]  Unit=1  AffineConversion=off
  Voltage Sensor2 : fl_lib/Electrical/Electrical Sensors/Voltage Sensor
  + : PMIOPort  Side=Left
  - : PMIOPort  Port=2  Side=Right
  tag scope: BCap=global
  wires:
  PS-Simulink Converter7/1 -> [BCap]
  connections:
  PS-Simulink Converter7/LConn1 -- Voltage Sensor2/RConn1
  Voltage Sensor2/LConn1 -- +/RConn1
  Voltage Sensor2/RConn2 -- -/RConn1

== system Modular_Model_New_Board/Module 3/Subsystem4 ==
  Current Sensor4 : fl_lib/Electrical/Electrical Sensors/Current Sensor
  PS-Simulink Converter6 : nesl_utility/PS-Simulink Converter  PhysicalDomain=network_engine_domain  SubClassName=ps_output  LeftPortType=input  RightPortType=output  PseudoPeriodic=off  Frequencies=[]  Unit=1  AffineConversion=off
  + : PMIOPort  Side=Left
  - : PMIOPort  Port=2  Side=Right
  tag scope: CCapCurr=global
  wires:
  PS-Simulink Converter6/1 -> [CCapCurr]
  connections:
  Current Sensor4/LConn1 -- +/RConn1
  PS-Simulink Converter6/LConn1 -- Current Sensor4/RConn1
  -/RConn1 -- Current Sensor4/RConn2

== system Modular_Model_New_Board/Module 3/Subsystem5 ==
  PS-Simulink Converter8 : nesl_utility/PS-Simulink Converter  PhysicalDomain=network_engine_domain  SubClassName=ps_output  LeftPortType=input  RightPortType=output  PseudoPeriodic=off  Frequencies=[]  Unit=1  AffineConversion=off
  Voltage Sensor4 : fl_lib/Electrical/Electrical Sensors/Voltage Sensor
  + : PMIOPort  Side=Left
  - : PMIOPort  Port=2  Side=Right
  tag scope: CCap=global
  wires:
  PS-Simulink Converter8/1 -> [CCap]
  connections:
  PS-Simulink Converter8/LConn1 -- Voltage Sensor4/RConn1
  Voltage Sensor4/LConn1 -- +/RConn1
  Voltage Sensor4/RConn2 -- -/RConn1

== system Modular_Model_New_Board/Module 3/Subsystem6 ==
  Current Sensor5 : fl_lib/Electrical/Electrical Sensors/Current Sensor
  PS-Simulink Converter9 : nesl_utility/PS-Simulink Converter  PhysicalDomain=network_engine_domain  SubClassName=ps_output  LeftPortType=input  RightPortType=output  PseudoPeriodic=off  Frequencies=[]  Unit=1  AffineConversion=off
  + : PMIOPort  Side=Left
  - : PMIOPort  Port=2  Side=Right
  Out1 : Outport
  wires:
  PS-Simulink Converter9/1 -> Out1/1
  connections:
  PS-Simulink Converter9/LConn1 -- Current Sensor5/RConn1
  Current Sensor5/LConn1 -- +/RConn1
  Current Sensor5/RConn2 -- -/RConn1

== system Modular_Model_New_Board/Module 3/Subsystem7 ==
  PS-Simulink Converter10 : nesl_utility/PS-Simulink Converter  PhysicalDomain=network_engine_domain  SubClassName=ps_output  LeftPortType=input  RightPortType=output  PseudoPeriodic=off  Frequencies=[]  Unit=1  AffineConversion=off
  Voltage Sensor5 : fl_lib/Electrical/Electrical Sensors/Voltage Sensor
  - : PMIOPort  Side=Right
  + : PMIOPort  Port=2  Side=Left
  Out1 : Outport
  wires:
  PS-Simulink Converter10/1 -> Out1/1
  connections:
  Voltage Sensor5/LConn1 -- +/RConn1
  Voltage Sensor5/RConn1 -- PS-Simulink Converter10/LConn1
  -/RConn1 -- Voltage Sensor5/RConn2

== system Modular_Model_New_Board/Module 3/Gate Driver10/Current Measure ==
  Current Sensor1 : fl_lib/Electrical/Electrical Sensors/Current Sensor
  PS-Simulink Converter4 : nesl_utility/PS-Simulink Converter  PhysicalDomain=network_engine_domain  SubClassName=ps_output  LeftPortType=input  RightPortType=output  PseudoPeriodic=off  Frequencies=[]  Unit=1  AffineConversion=off
  I+ : PMIOPort  Side=Left
  I- : PMIOPort  Port=2  Side=Right
  Data : Outport
  wires:
  PS-Simulink Converter4/1 -> Data/1
  connections:
  Current Sensor1/RConn2 -- I-/RConn1
  PS-Simulink Converter4/LConn1 -- Current Sensor1/RConn1
  Current Sensor1/LConn1 -- I+/RConn1

== system Modular_Model_New_Board/Module 3/Gate Driver10/Rate Limiter2 ==
  Inp : Inport
  Constant2 : Constant  Value=(VpulseMax - VpulseMin)/1e-9
  Constant3 : Constant  Value=(VpulseMin - VpulseMax)/1e-9
  Rate Limiter Dynamic : simulink/Discontinuities/Rate Limiter Dynamic
      settings: SourceProductName=Simulink
  Outp : Outport
  wires:
  Constant3/1 -> Rate Limiter Dynamic/3
  Constant2/1 -> Rate Limiter Dynamic/1
  Inp/1 -> Rate Limiter Dynamic/2
  Rate Limiter Dynamic/1 -> Outp/1

== system Modular_Model_New_Board/Module 3/Gate Driver10/Voltage Measure3 ==
  PS-Simulink Converter2 : nesl_utility/PS-Simulink Converter  PhysicalDomain=network_engine_domain  SubClassName=ps_output  LeftPortType=input  RightPortType=output  PseudoPeriodic=off  Frequencies=[]  Unit=1  AffineConversion=off
  Voltage Sensor3 : fl_lib/Electrical/Electrical Sensors/Voltage Sensor
  V+ : PMIOPort  Side=Right
  V- : PMIOPort  Port=2  Side=Right
  Data : Outport
  wires:
  PS-Simulink Converter2/1 -> Data/1
  connections:
  Voltage Sensor3/LConn1 -- V+/RConn1
  Voltage Sensor3/RConn2 -- V-/RConn1
  PS-Simulink Converter2/LConn1 -- Voltage Sensor3/RConn1

== system Modular_Model_New_Board/Module 3/Gate Driver11/Current Measure ==
  Current Sensor1 : fl_lib/Electrical/Electrical Sensors/Current Sensor
  PS-Simulink Converter4 : nesl_utility/PS-Simulink Converter  PhysicalDomain=network_engine_domain  SubClassName=ps_output  LeftPortType=input  RightPortType=output  PseudoPeriodic=off  Frequencies=[]  Unit=1  AffineConversion=off
  I+ : PMIOPort  Side=Left
  I- : PMIOPort  Port=2  Side=Right
  Data : Outport
  wires:
  PS-Simulink Converter4/1 -> Data/1
  connections:
  Current Sensor1/RConn2 -- I-/RConn1
  PS-Simulink Converter4/LConn1 -- Current Sensor1/RConn1
  Current Sensor1/LConn1 -- I+/RConn1

== system Modular_Model_New_Board/Module 3/Gate Driver11/Rate Limiter2 ==
  Inp : Inport
  Constant2 : Constant  Value=(VpulseMax - VpulseMin)/1e-9
  Constant3 : Constant  Value=(VpulseMin - VpulseMax)/1e-9
  Rate Limiter Dynamic : simulink/Discontinuities/Rate Limiter Dynamic
      settings: SourceProductName=Simulink
  Outp : Outport
  wires:
  Constant3/1 -> Rate Limiter Dynamic/3
  Constant2/1 -> Rate Limiter Dynamic/1
  Inp/1 -> Rate Limiter Dynamic/2
  Rate Limiter Dynamic/1 -> Outp/1

== system Modular_Model_New_Board/Module 3/Gate Driver11/Voltage Measure3 ==
  PS-Simulink Converter2 : nesl_utility/PS-Simulink Converter  PhysicalDomain=network_engine_domain  SubClassName=ps_output  LeftPortType=input  RightPortType=output  PseudoPeriodic=off  Frequencies=[]  Unit=1  AffineConversion=off
  Voltage Sensor3 : fl_lib/Electrical/Electrical Sensors/Voltage Sensor
  V+ : PMIOPort  Side=Right
  V- : PMIOPort  Port=2  Side=Right
  Data : Outport
  wires:
  PS-Simulink Converter2/1 -> Data/1
  connections:
  Voltage Sensor3/LConn1 -- V+/RConn1
  Voltage Sensor3/RConn2 -- V-/RConn1
  PS-Simulink Converter2/LConn1 -- Voltage Sensor3/RConn1

== system Modular_Model_New_Board/Module 3/Gate Driver6/Current Measure ==
  Current Sensor1 : fl_lib/Electrical/Electrical Sensors/Current Sensor
  PS-Simulink Converter4 : nesl_utility/PS-Simulink Converter  PhysicalDomain=network_engine_domain  SubClassName=ps_output  LeftPortType=input  RightPortType=output  PseudoPeriodic=off  Frequencies=[]  Unit=1  AffineConversion=off
  I+ : PMIOPort  Side=Left
  I- : PMIOPort  Port=2  Side=Right
  Data : Outport
  wires:
  PS-Simulink Converter4/1 -> Data/1
  connections:
  Current Sensor1/RConn2 -- I-/RConn1
  PS-Simulink Converter4/LConn1 -- Current Sensor1/RConn1
  Current Sensor1/LConn1 -- I+/RConn1

== system Modular_Model_New_Board/Module 3/Gate Driver6/Rate Limiter2 ==
  Inp : Inport
  Constant2 : Constant  Value=(VpulseMax - VpulseMin)/1e-9
  Constant3 : Constant  Value=(VpulseMin - VpulseMax)/1e-9
  Rate Limiter Dynamic : simulink/Discontinuities/Rate Limiter Dynamic
      settings: SourceProductName=Simulink
  Outp : Outport
  wires:
  Constant3/1 -> Rate Limiter Dynamic/3
  Constant2/1 -> Rate Limiter Dynamic/1
  Inp/1 -> Rate Limiter Dynamic/2
  Rate Limiter Dynamic/1 -> Outp/1

== system Modular_Model_New_Board/Module 3/Gate Driver6/Voltage Measure3 ==
  PS-Simulink Converter2 : nesl_utility/PS-Simulink Converter  PhysicalDomain=network_engine_domain  SubClassName=ps_output  LeftPortType=input  RightPortType=output  PseudoPeriodic=off  Frequencies=[]  Unit=1  AffineConversion=off
  Voltage Sensor3 : fl_lib/Electrical/Electrical Sensors/Voltage Sensor
  V+ : PMIOPort  Side=Right
  V- : PMIOPort  Port=2  Side=Right
  Data : Outport
  wires:
  PS-Simulink Converter2/1 -> Data/1
  connections:
  Voltage Sensor3/LConn1 -- V+/RConn1
  Voltage Sensor3/RConn2 -- V-/RConn1
  PS-Simulink Converter2/LConn1 -- Voltage Sensor3/RConn1

== system Modular_Model_New_Board/Module 3/Gate Driver7/Current Measure ==
  Current Sensor1 : fl_lib/Electrical/Electrical Sensors/Current Sensor
  PS-Simulink Converter4 : nesl_utility/PS-Simulink Converter  PhysicalDomain=network_engine_domain  SubClassName=ps_output  LeftPortType=input  RightPortType=output  PseudoPeriodic=off  Frequencies=[]  Unit=1  AffineConversion=off
  I+ : PMIOPort  Side=Left
  I- : PMIOPort  Port=2  Side=Right
  Data : Outport
  wires:
  PS-Simulink Converter4/1 -> Data/1
  connections:
  Current Sensor1/RConn2 -- I-/RConn1
  PS-Simulink Converter4/LConn1 -- Current Sensor1/RConn1
  Current Sensor1/LConn1 -- I+/RConn1

== system Modular_Model_New_Board/Module 3/Gate Driver7/Rate Limiter2 ==
  Inp : Inport
  Constant2 : Constant  Value=(VpulseMax - VpulseMin)/1e-9
  Constant3 : Constant  Value=(VpulseMin - VpulseMax)/1e-9
  Rate Limiter Dynamic : simulink/Discontinuities/Rate Limiter Dynamic
      settings: SourceProductName=Simulink
  Outp : Outport
  wires:
  Constant3/1 -> Rate Limiter Dynamic/3
  Constant2/1 -> Rate Limiter Dynamic/1
  Inp/1 -> Rate Limiter Dynamic/2
  Rate Limiter Dynamic/1 -> Outp/1

== system Modular_Model_New_Board/Module 3/Gate Driver7/Voltage Measure3 ==
  PS-Simulink Converter2 : nesl_utility/PS-Simulink Converter  PhysicalDomain=network_engine_domain  SubClassName=ps_output  LeftPortType=input  RightPortType=output  PseudoPeriodic=off  Frequencies=[]  Unit=1  AffineConversion=off
  Voltage Sensor3 : fl_lib/Electrical/Electrical Sensors/Voltage Sensor
  V+ : PMIOPort  Side=Right
  V- : PMIOPort  Port=2  Side=Right
  Data : Outport
  wires:
  PS-Simulink Converter2/1 -> Data/1
  connections:
  Voltage Sensor3/LConn1 -- V+/RConn1
  Voltage Sensor3/RConn2 -- V-/RConn1
  PS-Simulink Converter2/LConn1 -- Voltage Sensor3/RConn1

== system Modular_Model_New_Board/Module 3/Gate Driver8/Current Measure ==
  Current Sensor1 : fl_lib/Electrical/Electrical Sensors/Current Sensor
  PS-Simulink Converter4 : nesl_utility/PS-Simulink Converter  PhysicalDomain=network_engine_domain  SubClassName=ps_output  LeftPortType=input  RightPortType=output  PseudoPeriodic=off  Frequencies=[]  Unit=1  AffineConversion=off
  I+ : PMIOPort  Side=Left
  I- : PMIOPort  Port=2  Side=Right
  Data : Outport
  wires:
  PS-Simulink Converter4/1 -> Data/1
  connections:
  Current Sensor1/RConn2 -- I-/RConn1
  PS-Simulink Converter4/LConn1 -- Current Sensor1/RConn1
  Current Sensor1/LConn1 -- I+/RConn1

== system Modular_Model_New_Board/Module 3/Gate Driver8/Rate Limiter2 ==
  Inp : Inport
  Constant2 : Constant  Value=(VpulseMax - VpulseMin)/1e-9
  Constant3 : Constant  Value=(VpulseMin - VpulseMax)/1e-9
  Rate Limiter Dynamic : simulink/Discontinuities/Rate Limiter Dynamic
      settings: SourceProductName=Simulink
  Outp : Outport
  wires:
  Constant3/1 -> Rate Limiter Dynamic/3
  Constant2/1 -> Rate Limiter Dynamic/1
  Inp/1 -> Rate Limiter Dynamic/2
  Rate Limiter Dynamic/1 -> Outp/1

== system Modular_Model_New_Board/Module 3/Gate Driver8/Voltage Measure3 ==
  PS-Simulink Converter2 : nesl_utility/PS-Simulink Converter  PhysicalDomain=network_engine_domain  SubClassName=ps_output  LeftPortType=input  RightPortType=output  PseudoPeriodic=off  Frequencies=[]  Unit=1  AffineConversion=off
  Voltage Sensor3 : fl_lib/Electrical/Electrical Sensors/Voltage Sensor
  V+ : PMIOPort  Side=Right
  V- : PMIOPort  Port=2  Side=Right
  Data : Outport
  wires:
  PS-Simulink Converter2/1 -> Data/1
  connections:
  Voltage Sensor3/LConn1 -- V+/RConn1
  Voltage Sensor3/RConn2 -- V-/RConn1
  PS-Simulink Converter2/LConn1 -- Voltage Sensor3/RConn1

== system Modular_Model_New_Board/Module 3/Gate Driver9/Current Measure ==
  Current Sensor1 : fl_lib/Electrical/Electrical Sensors/Current Sensor
  PS-Simulink Converter4 : nesl_utility/PS-Simulink Converter  PhysicalDomain=network_engine_domain  SubClassName=ps_output  LeftPortType=input  RightPortType=output  PseudoPeriodic=off  Frequencies=[]  Unit=1  AffineConversion=off
  I+ : PMIOPort  Side=Left
  I- : PMIOPort  Port=2  Side=Right
  Data : Outport
  wires:
  PS-Simulink Converter4/1 -> Data/1
  connections:
  Current Sensor1/RConn2 -- I-/RConn1
  PS-Simulink Converter4/LConn1 -- Current Sensor1/RConn1
  Current Sensor1/LConn1 -- I+/RConn1

== system Modular_Model_New_Board/Module 3/Gate Driver9/Rate Limiter2 ==
  Inp : Inport
  Constant2 : Constant  Value=(VpulseMax - VpulseMin)/1e-9
  Constant3 : Constant  Value=(VpulseMin - VpulseMax)/1e-9
  Rate Limiter Dynamic : simulink/Discontinuities/Rate Limiter Dynamic
      settings: SourceProductName=Simulink
  Outp : Outport
  wires:
  Constant3/1 -> Rate Limiter Dynamic/3
  Constant2/1 -> Rate Limiter Dynamic/1
  Inp/1 -> Rate Limiter Dynamic/2
  Rate Limiter Dynamic/1 -> Outp/1

== system Modular_Model_New_Board/Module 3/Gate Driver9/Voltage Measure3 ==
  PS-Simulink Converter2 : nesl_utility/PS-Simulink Converter  PhysicalDomain=network_engine_domain  SubClassName=ps_output  LeftPortType=input  RightPortType=output  PseudoPeriodic=off  Frequencies=[]  Unit=1  AffineConversion=off
  Voltage Sensor3 : fl_lib/Electrical/Electrical Sensors/Voltage Sensor
  V+ : PMIOPort  Side=Right
  V- : PMIOPort  Port=2  Side=Right
  Data : Outport
  wires:
  PS-Simulink Converter2/1 -> Data/1
  connections:
  Voltage Sensor3/LConn1 -- V+/RConn1
  Voltage Sensor3/RConn2 -- V-/RConn1
  PS-Simulink Converter2/LConn1 -- Voltage Sensor3/RConn1

== system Modular_Model_New_Board/Module 3/R L Load2/Current Measure1 ==
  Current Sensor1 : fl_lib/Electrical/Electrical Sensors/Current Sensor
  PS-Simulink Converter4 : nesl_utility/PS-Simulink Converter  PhysicalDomain=network_engine_domain  SubClassName=ps_output  LeftPortType=input  RightPortType=output  PseudoPeriodic=off  Frequencies=[]  Unit=1  AffineConversion=off
  I+ : PMIOPort  Side=Left
  I- : PMIOPort  Port=2  Side=Right
  Data : Outport
  wires:
  PS-Simulink Converter4/1 -> Data/1
  connections:
  Current Sensor1/LConn1 -- I+/RConn1
  PS-Simulink Converter4/LConn1 -- Current Sensor1/RConn1
  Current Sensor1/RConn2 -- I-/RConn1

== system Modular_Model_New_Board/Module 3/R L Load2/Current Measure2 ==
  Current Sensor1 : fl_lib/Electrical/Electrical Sensors/Current Sensor
  PS-Simulink Converter4 : nesl_utility/PS-Simulink Converter  PhysicalDomain=network_engine_domain  SubClassName=ps_output  LeftPortType=input  RightPortType=output  PseudoPeriodic=off  Frequencies=[]  Unit=1  AffineConversion=off
  I+ : PMIOPort  Side=Left
  I- : PMIOPort  Port=2  Side=Right
  Data : Outport
  wires:
  PS-Simulink Converter4/1 -> Data/1
  connections:
  Current Sensor1/RConn2 -- I-/RConn1
  PS-Simulink Converter4/LConn1 -- Current Sensor1/RConn1
  Current Sensor1/LConn1 -- I+/RConn1

== system Modular_Model_New_Board/Module 3/R L Load2/Current Measure5 ==
  Current Sensor1 : fl_lib/Electrical/Electrical Sensors/Current Sensor
  PS-Simulink Converter4 : nesl_utility/PS-Simulink Converter  PhysicalDomain=network_engine_domain  SubClassName=ps_output  LeftPortType=input  RightPortType=output  PseudoPeriodic=off  Frequencies=[]  Unit=1  AffineConversion=off
  I+ : PMIOPort  Side=Left
  I- : PMIOPort  Port=2  Side=Right
  Data : Outport
  wires:
  PS-Simulink Converter4/1 -> Data/1
  connections:
  Current Sensor1/RConn2 -- I-/RConn1
  PS-Simulink Converter4/LConn1 -- Current Sensor1/RConn1
  Current Sensor1/LConn1 -- I+/RConn1

== system Modular_Model_New_Board/Module 3/R L Load2/Voltage Measure1 ==
  PS-Simulink Converter2 : nesl_utility/PS-Simulink Converter  PhysicalDomain=network_engine_domain  SubClassName=ps_output  LeftPortType=input  RightPortType=output  PseudoPeriodic=off  Frequencies=[]  Unit=1  AffineConversion=off
  Voltage Sensor3 : fl_lib/Electrical/Electrical Sensors/Voltage Sensor
  V+ : PMIOPort  Side=Right
  V- : PMIOPort  Port=2  Side=Right
  Data : Outport
  wires:
  PS-Simulink Converter2/1 -> Data/1
  connections:
  PS-Simulink Converter2/LConn1 -- Voltage Sensor3/RConn1
  Voltage Sensor3/RConn2 -- V-/RConn1
  Voltage Sensor3/LConn1 -- V+/RConn1

== system Modular_Model_New_Board/Module 3/R L Load2/Voltage Measure3 ==
  PS-Simulink Converter2 : nesl_utility/PS-Simulink Converter  PhysicalDomain=network_engine_domain  SubClassName=ps_output  LeftPortType=input  RightPortType=output  PseudoPeriodic=off  Frequencies=[]  Unit=1  AffineConversion=off
  Voltage Sensor3 : fl_lib/Electrical/Electrical Sensors/Voltage Sensor
  V+ : PMIOPort  Side=Right
  V- : PMIOPort  Port=2  Side=Right
  Data : Outport
  wires:
  PS-Simulink Converter2/1 -> Data/1
  connections:
  Voltage Sensor3/LConn1 -- V+/RConn1
  Voltage Sensor3/RConn2 -- V-/RConn1
  PS-Simulink Converter2/LConn1 -- Voltage Sensor3/RConn1

== system Modular_Model_New_Board/Module 3/R L Load2/Voltage Measure4 ==
  PS-Simulink Converter2 : nesl_utility/PS-Simulink Converter  PhysicalDomain=network_engine_domain  SubClassName=ps_output  LeftPortType=input  RightPortType=output  PseudoPeriodic=off  Frequencies=[]  Unit=1  AffineConversion=off
  Voltage Sensor3 : fl_lib/Electrical/Electrical Sensors/Voltage Sensor
  V+ : PMIOPort  Side=Right
  V- : PMIOPort  Port=2  Side=Right
  Data : Outport
  wires:
  PS-Simulink Converter2/1 -> Data/1
  connections:
  PS-Simulink Converter2/LConn1 -- Voltage Sensor3/RConn1
  Voltage Sensor3/RConn2 -- V-/RConn1
  Voltage Sensor3/LConn1 -- V+/RConn1
